simulink model "VFM_linecut_exp"  (R2025a)
settings: Solver=FixedStepAuto  StartTime=0.0  StopTime=t_end+t_sim_start  FixedStep=Ts  RelTol=1e-3
InitFcn:
  | run VFMPara_exp.m
values from neighbouring files (symbols this model uses):
  Cf = 0.0083    [GFMPara.m]    (also in GFMPara_exp.m = 0.0249; VFMPara.m = 0.02; VFMPara_exp.m = 0.03)
  dt_sag = t_c    [GFMPara.m]    (also in GFMPara_exp.m; PLLpara.m; VFMPara.m; VFMPara_exp.m)
  f_switching = 20e3    (= 20000)    [GFMPara_exp.m]    (also in PLLpara.m = 10000; VFMPara_exp.m)
  Lc = 1e-9    (= 1e-09)    [GFMPara.m]    (also in GFMPara_exp.m; PLLpara.m; VFMPara.m; VFMPara_exp.m)
  Lf = 0.0592    [GFMPara.m]    (also in GFMPara_exp.m; PLLpara.m = 0.05; VFMPara.m = 0.05; VFMPara_exp.m = 0.05)
  Lg1 = X1    [PLLpara.m]    (also in VFMPara.m; VFMPara_exp.m)
  Lgg = Xgg    [PLLpara.m]    (also in VFMPara.m; VFMPara_exp.m)
  m_gfm = 1/D    [GFMPara.m]    (also in GFMPara_exp.m)
  Rf = 1e-3    (= 0.001)    [PLLpara.m]
  Rg1 = R1    [PLLpara.m]    (also in VFMPara.m; VFMPara_exp.m = 4*R1/5)
  Rgg = Rgg    [PLLpara.m]    (also in VFMPara.m; VFMPara_exp.m)
  Sbase = 1    [GFMPara.m]    (also in GFMPara_exp.m; PLLpara.m; VFMPara.m; VFMPara_exp.m)
  Scale_ki_v = 20    [GFMPara.m]    (also in GFMPara_exp.m; VFMPara.m; VFMPara_exp.m)
  t0 = t_sim_start +t_start    [PLLpara.m]    (also in VFMPara_exp.m)
  t0_sag = t_sim_start +t_start    [GFMPara.m]    (also in GFMPara_exp.m; PLLpara.m = 20; VFMPara.m; VFMPara_exp.m = 20)
  tc = t_c    [PLLpara.m]    (also in VFMPara_exp.m)
  Tc = 1/f_switching    (= 5e-05)    [GFMPara_exp.m]    (also in PLLpara.m = 0.0001; VFMPara_exp.m)
  Ts = 1/Fs    (= 1e-05)    [GFMPara.m]    (also in GFMPara_exp.m = 1e-06; PLLpara.m = 1e-06; VFMPara.m = 5e-06; VFMPara_exp.m = 1e-06)
  v_sag = Ug_fault    [GFMPara.m]    (also in GFMPara_exp.m; PLLpara.m; VFMPara.m; VFMPara_exp.m)
  Vbase = 1    [GFMPara.m]    (also in GFMPara_exp.m; PLLpara.m; VFMPara.m; VFMPara_exp.m)
  Vdc = 2.5    [PLLpara.m]
  Vdc_ref = 2.5    [GFMPara_exp.m]
  w_droop = D/J    [GFMPara.m]    (also in GFMPara_exp.m; VFMPara.m = 314.159265359; VFMPara_exp.m = 314.159265359)
  w_i_GFM = 2000*2*pi    (= 12566.3706144)    [GFMPara.m]    (also in GFMPara_exp.m = 9424.77796077; VFMPara.m = 9424.77796077; VFMPara_exp.m = 9424.77796077)
  w_v_GFM = 800 *2*pi    (= 5026.54824574)    [GFMPara.m]    (also in GFMPara_exp.m = 3141.59265359; VFMPara.m = 3141.59265359; VFMPara_exp.m = 3141.59265359)
  Wbase = 2*pi*50    (= 314.159265359)    [GFMPara.m]    (also in GFMPara_exp.m; PLLpara.m; VFMPara.m; VFMPara_exp.m)
  Zbase = Vbase/Ibase    (= 1)    [GFMPara.m]    (also in GFMPara_exp.m; PLLpara.m; VFMPara.m; VFMPara_exp.m)
undefined symbols (not defined in the file or in its folder): DiscIntNeverNeededParam, dspblkCoreblockFVToolHelper, gcbh, initial, Kip, Kpp, Pin, Ws, Y_dc
libraries: spsVoltageMeasurementLib x51, spsCurrentMeasurementLib x48, spsThreePhaseSeriesRLCBranchLib x14, spsControlledVoltageSourceLib x9, spsSeriesRLCBranchLib x8, spsIdealSwitchLib x7, simulink x6, spsThreePhaseBreakerLib x4, spsDCVoltageSourceLib x4, spsControlledCurrentSourceLib x3, spsDiodeLib x3, spsHalfBridgeConverterLib x3
(part 2 of 4)

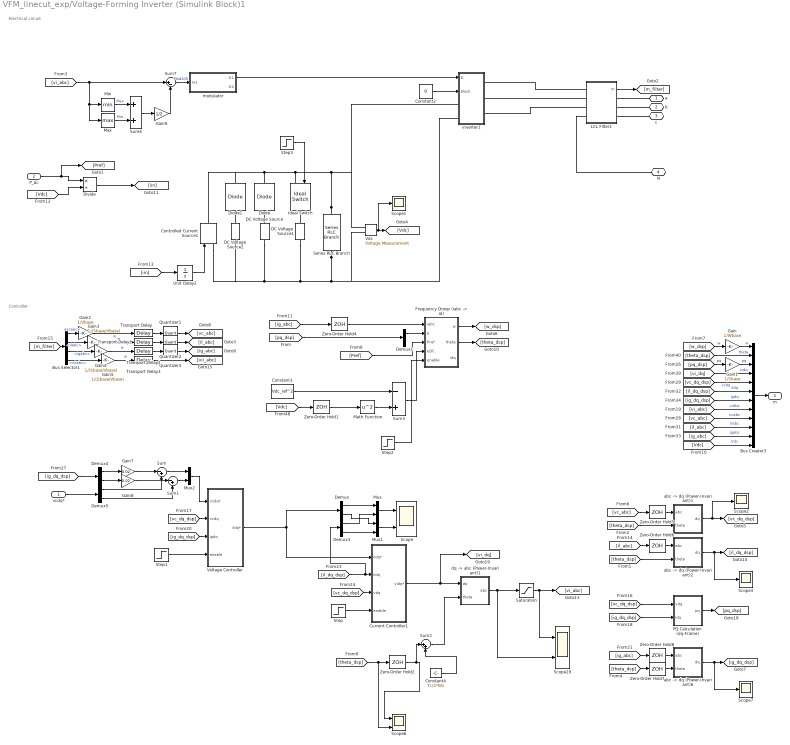
== system VFM_linecut_exp/Voltage-Forming Inverter (Simulink Block)1 ==
  note: Controller
  note: Electrical circuit
  vcdq* : Inport
  P_dc : Inport  Port=2
  Bus Creator3 : BusCreator  Inputs=12
  Bus Selector1 : BusSelector  OutputSignals=vcabc,ilabc,igabc,viiabc
  Constant2 : Constant  Value=0
  Constant3 : Constant  Value=Vdc_ref^2
  Constant4 : Constant  Value=Tc/2*Ws
  Controlled Current Source1 : spsControlledCurrentSourceLib/Controlled Current Source  Initialize=on  Source_Type=AC  Amplitude=0  Phase=0  Frequency=0  Measurements=None
  Current Controller1 : Subsystem  mask{Ts=Tc, Wbase=Wbase, Lf=Lf/Wbase, Kg=0, Kp=w_i*Lf/Wbase*1.5, Ki=w_i*w_i/4*Lf/Wbase, vdmax=Vdc/sqrt(2), vqmax=Vdc/sqrt(2), Kcd=0, Kic=0}
      mask prompts: Ts "Sampling Time (s)"; Wbase "Base Angular Frequency (rad/s)"; Lf "Inductance"; Kg "Estimator Gain"; Kp "Proportional Gain"; Ki "Integral Gain"; vdmax "Voltage D Limit"; vqmax "Voltage Q Limit"; Kcd "Cross Decoupling Gain"; Kic "Capacitor Current Gain"
  DC Voltage Source : spsDCVoltageSourceLib/DC Voltage Source  Amplitude=3.25  Measurements=None
  DC Voltage Source1 : spsDCVoltageSourceLib/DC Voltage Source  Amplitude=2.5  Measurements=None
  DC Voltage Source2 : spsDCVoltageSourceLib/DC Voltage Source  Amplitude=2  Measurements=None
  Demux{,1,3..5} (5 alike) : Demux  Outputs=2
  Diode : spsDiodeLib/Diode  Ron=0.01  Lon=0  Vf=0  IC=0  UseSnubber=0  Rs=1e6  Cs=inf  Measurements=off
  Diode1 : spsDiodeLib/Diode  Ron=0.01  Lon=0  Vf=0  IC=0  UseSnubber=0  Rs=1e6  Cs=inf  Measurements=off
  Divide : Product  Inputs=*/
  "Frequency Droop (iabc -> id)" : Subsystem  AncestorBlock=|  mask{Ts=Tc, Sbase=Sbase, Vbase=Vbase, Wbase=Wbase, m=m, w_tau=w_droop, theta0=0, i0=Pin, w0=1}
      | SimplexPS/Frequency Droop
      | (iabc -> id)
      mask prompts: Ts "Ts (s), samping period"; Sbase "Sbase (VA), base power"; Vbase "Vbase (V), base voltage"; Wbase "Wbase (rad/s), base angular frequency"; m "m (pu), droop gain"; w_tau "w_tau (rad/s), low-pass filter bandwidth"; theta0 "theta0 (rad), initial angle"; i0 "i0 (pu), current setting point"; w0 "w0 (pu), frequency setting point"
  Gain : Gain  Gain=1/Wbase
  Gain1 : Gain  Gain=1/Sbase
  Gain2 : Gain  Gain=1/Vbase
  Gain3 : Gain  Gain=1/(Sbase/Vbase)
  Gain4 : Gain  Gain=1/(Sbase/Vbase)
  Gain5 : Gain  Gain=1/(Sbase/Vbase)
  Gain7 : Gain  Gain=0.02
  Gain8 : Gain  Gain=0.02
  Gain9 : Gain  Gain=1/2
  Ideal Switch : spsIdealSwitchLib/Ideal Switch  Ron=0.001  Lon=0  IC=0  Rs=1e8  Cs=inf  Measurements=off
  LCL Filter1 : Subsystem  mask{Lf=Lf*(Vbase^2/Sbase)/Wbase, Rf=Lf*(Vbase^2/Sbase)*2e-6, Lc=1e-9*(Vbase^2/Sbase)/Wbase, Rc=1e-9*(Vbase^2/Sbase), Cf=Cf*(Sbase/Vbase^2)/Wbase, Rd=1e-3*(Vbase^2/Sbase)}
      mask prompts: Lf "Lf (H)"; Rf "Rf (Ohm)"; Lc "Lc (H)"; Rc "Rc (Ohm)"; Cf "Cf (F)"; Rd "Rd (Ohm)"
  Math Function : Math  Operator=square
  Max : MinMax  Function=max
  Min : MinMax
  Mux : Mux  Inputs=2
  Mux1 : Mux  Inputs=2
  Mux2 : Mux  Inputs=2
  PQ Calculation (dq-Frame) : Subsystem
  Quantizer1 : Quantizer  QuantizationInterval=5/4095
  Quantizer2 : Quantizer  QuantizationInterval=5/4095
  Quantizer3 : Quantizer  QuantizationInterval=5/4095
  Saturation : Saturate  UpperLimit=Vdc_ref/sqrt(3)  LowerLimit=-Vdc_ref/sqrt(3)
  Scope : Scope  NumInputPorts=2
      settings: ActiveDisplayYMinimum=-2.0933971200476993  ActiveDisplayYMaximum=2.0858879407185071  DataLoggingVariableName=ScopeData4
  Scope{1..3,7} (4 alike) : Scope
      Scope1 settings: ActiveDisplayYMinimum=2.0924827237669028  ActiveDisplayYMaximum=4.2567675140943511  DataLoggingVariableName=ScopeData8
      Scope2 settings: ActiveDisplayYMinimum=-2.4523  ActiveDisplayYMaximum=2.43362  DataLoggingVariableName=ScopeData9
      Scope3 settings: ActiveDisplayYMinimum=0.94065  ActiveDisplayYMaximum=1.03256  DataLoggingVariableName=ScopeData11
      Scope7 settings: ActiveDisplayYMinimum=-0.01957  ActiveDisplayYMaximum=0.02954  DataLoggingVariableName=ScopeData10
  Scope29 : Scope  NumInputPorts=2
      settings: ActiveDisplayYMinimum=-28.9342  ActiveDisplayYMaximum=29.0712  DataLoggingVariableName=ScopeData14
  Scope6 : Scope  NumInputPorts=2
      settings: ActiveDisplayYMinimum=2.25613  ActiveDisplayYMaximum=3.2738  DataLoggingVariableName=ScopeData16
  Series RLC Branch : spsSeriesRLCBranchLib/Series RLC Branch  LConnTagsString=__new0  RConnTagsString=__new0  BranchType=RC  Resistance=1e-10*(Vbase^2/Sbase)  Inductance=1e-3  SetiL0=off  InitialCurrent=0  Capacitance=Y_dc*(Sbase/Vbase^2)/Wbase  Setx0=on  InitialVoltage=Vdc_ref  Measurements=None
  Step : Step  Time=0.1  SampleTime=0
  Step1 : Step  Time=0.1  SampleTime=0
  Step2 : Step  Time=0.1  SampleTime=0
  Step3 : Step  Time=0.1  Before=1  After=0  SampleTime=0
  Sum : Sum  Inputs=|-+
  Sum1 : Sum  Inputs=|-+
  Sum2 : Sum  Inputs=|++  InputSameDT=on  SaturateOnIntegerOverflow=on  OutDataTypeStr=Inherit: Same as first input
  Sum3 : Sum  Inputs=-+
  Sum6 : Sum  InputSameDT=on  SaturateOnIntegerOverflow=on  OutDataTypeStr=Inherit: Same as first input
  Sum7 : Sum  Inputs=|+-  InputSameDT=on  SaturateOnIntegerOverflow=on  OutDataTypeStr=Inherit: Same as first input
  Transport Delay{,1..3} (4 alike) : TransportDelay  DelayTime=6e-6
  Unit Delay2 : UnitDelay  SampleTime=-1  HasFrameUpgradeWarning=on
  Vdc : spsVoltageMeasurementLib/Voltage Measurement  PhasorSimulation=off  OutputType=Complex  PSBequivalent=0
  Voltage Controller : Subsystem  mask{Ts=Tc, Wbase=Wbase, Cf=Cf/Wbase, Kg=0, Kp=w_v*Cf/Wbase, Ki=w_v*w_v/4*Cf/Wbase*Scale_ki_v, xdmax=inf, xqmax=inf, Kcd=0}
      mask prompts: Ts "Sampling Time (s)"; Wbase "Base Angular Frequency (rad/s)"; Cf "Capacitance"; Kg "Estimator Gain"; Kp "Proportional Gain"; Ki "Integral Gain"; xdmax "Current D Limit"; xqmax "Current Q Limit"; Kcd "Cross Decoupling Gain"
  Zero-Order Hold{1..2,4..8} (7 alike) : ZeroOrderHold  SampleTime=Tc
  "abc -> dq (Power-Invariant)1" : Subsystem  AncestorBlock=|
      | SimplusGT/abc -> dq
      | (Power-Invariant)
  "abc -> dq (Power-Invariant)2" : Subsystem  AncestorBlock=|
      | SimplusGT/abc -> dq
      | (Power-Invariant)
  "abc -> dq (Power-Invariant)6" : Subsystem  AncestorBlock=|
      | SimplusGT/abc -> dq
      | (Power-Invariant)
  "dq -> abc (Power-Invariant)1" : Subsystem  AncestorBlock=|
      | SimplusGT/dq -> abc
      | (Power-Invariant)
  inverter1 : Subsystem
  modulator : Subsystem
  a : PMIOPort  Side=Right
  b : PMIOPort  Port=2  Side=Right
  c : PMIOPort  Port=3  Side=Right
  N : PMIOPort  Port=4  Side=Right
  m : Outport
  wires:
  [ig_abc] -> Bus Creator3/11  "igabc"
  [il_abc] -> Bus Creator3/10  "ilabc"
  [vc_abc] -> Bus Creator3/9  "vcabc"
  [vi_abc] -> Bus Creator3/8  "viabc"
  [ig_dq_dsp] -> Bus Creator3/7  "igdq"
  [il_dq_dsp] -> Bus Creator3/6  "ildq"
  [vc_dq_dsp] -> Bus Creator3/5  "vcdq"
  [vi_dq] -> Bus Creator3/4  "vidq"
  Gain1/1 -> Bus Creator3/3  "pq"
  [theta_dsp] -> Bus Creator3/2  "theta"
  Gain/1 -> Bus Creator3/1  "w"
  [pq_dsp] -> Gain1/1  "pq"
  [w_dsp] -> Gain/1  "w"
  [ig_abc] -> Zero-Order Hold4/1
  [ig_dq_dsp] -> PQ Calculation (dq-Frame)/2(idq)
  PQ Calculation (dq-Frame)/1(pq) -> [pq_dsp]
  [vc_dq_dsp] -> PQ Calculation (dq-Frame)/1(vdq)
  "Frequency Droop (iabc -> id)"/1(w) -> [w_dsp]
  "Frequency Droop (iabc -> id)"/2(theta) -> [theta_dsp]
  Bus Creator3/1 -> m/1
  Demux1/1 -> "Frequency Droop (iabc -> id)"/2(p)
  [pq_dsp] -> Demux1/1
  Bus Selector1/3 -> Gain4/1  "<igabc>"
  Bus Selector1/2 -> Gain3/1  "<ilabc>"
  Bus Selector1/1 -> Gain2/1  "<vcabc>"
  Gain4/1 -> Transport Delay2/1  "w"
  [m_filter] -> Bus Selector1/1
  Gain2/1 -> Transport Delay/1  "w"
  Gain3/1 -> Transport Delay1/1  "w"
  P_dc/1 -> [Pref], Divide/1
  Vdc/1 -> Scope1/1, [Vdc]
  [iin] -> Unit Delay2/1
  LCL Filter1/1(m) -> [m_filter]
  Divide/1 -> [iin]
  Unit Delay2/1 -> Controlled Current Source1/1
  [Vdc] -> Divide/2
  [Pref] -> "Frequency Droop (iabc -> id)"/3(Pref)
  Math Function/1 -> Sum3/2
  Constant3/1 -> Sum3/1
  [Vdc] -> Zero-Order Hold1/1
  Sum3/1 -> "Frequency Droop (iabc -> id)"/4(eDC)
  [Vdc] -> Bus Creator3/12  "Vdc"
  Step/1 -> Current Controller1/4(enable)
  Current Controller1/1(vidq*) -> "dq -> abc (Power-Invariant)1"/1(dq), [vi_dq]
  [vc_dq_dsp] -> Voltage Controller/2(vcdq)
  [vc_dq_dsp] -> Current Controller1/3(vdq)
  [il_dq_dsp] -> Current Controller1/2(iIdq), Demux3/1
  [ig_dq_dsp] -> Voltage Controller/3(igdq)
  "dq -> abc (Power-Invariant)1"/1(abc) -> Scope29/2, Saturation/1
  Sum2/1 -> "dq -> abc (Power-Invariant)1"/2(theta)
  Bus Selector1/4 -> Gain5/1  "<viiabc>"
  Gain5/1 -> Transport Delay3/1  "w"
  Mux/1 -> Scope/1
  Mux1/1 -> Scope/2
  Demux/1 -> Mux/1
  Demux3/1 -> Mux/2
  Demux/2 -> Mux1/1
  Demux3/2 -> Mux1/2
  Demux4/1 -> Gain7/1
  [ig_dq_dsp] -> Demux4/1
  vcdq*/1 -> Demux5/1
  Demux4/2 -> Gain8/1
  Gain8/1 -> Sum1/1
  Gain7/1 -> Sum/1
  Demux5/1 -> Sum/2
  Sum/1 -> Mux2/1
  Demux5/2 -> Sum1/2
  Sum1/1 -> Mux2/2
  Mux2/1 -> Voltage Controller/1(vcdq*)
  Sum7/1 -> modulator/1(In1)  "ModA/B"
  Sum6/1 -> Gain9/1
  [vi_abc] -> Sum7/1, Max/1, Min/1
  Max/1 -> Sum6/2  "Min"
  Gain9/1 -> Sum7/2
  Min/1 -> Sum6/1  "Max"
  modulator/1(G1) -> inverter1/1(G)
  Constant2/1 -> inverter1/2(block)
  Transport Delay/1 -> Quantizer1/1
  Transport Delay1/1 -> Quantizer2/1
  Transport Delay2/1 -> Quantizer3/1
  Transport Delay3/1 -> [vii_abc]
  Zero-Order Hold4/1 -> "Frequency Droop (iabc -> id)"/1(iabc)
  [il_abc] -> Zero-Order Hold6/1
  [theta_dsp] -> "abc -> dq (Power-Invariant)1"/2(theta)
  "abc -> dq (Power-Invariant)2"/1(dq) -> Scope3/1, [il_dq_dsp]
  Zero-Order Hold5/1 -> "abc -> dq (Power-Invariant)1"/1(abc)
  Zero-Order Hold6/1 -> "abc -> dq (Power-Invariant)2"/1(abc)
  [vc_abc] -> Zero-Order Hold5/1
  "abc -> dq (Power-Invariant)1"/1(dq) -> Scope2/1, [vc_dq_dsp]
  [theta_dsp] -> "abc -> dq (Power-Invariant)2"/2(theta)
  Zero-Order Hold7/1 -> "abc -> dq (Power-Invariant)6"/2(theta)
  [theta_dsp] -> Zero-Order Hold7/1
  "abc -> dq (Power-Invariant)6"/1(dq) -> Scope7/1, [ig_dq_dsp]
  Zero-Order Hold8/1 -> "abc -> dq (Power-Invariant)6"/1(abc)
  [ig_abc] -> Zero-Order Hold8/1
  Zero-Order Hold1/1 -> Math Function/1
  Saturation/1 -> Scope29/1, [vi_abc]
  [theta_dsp] -> Scope6/2, Zero-Order Hold2/1
  Zero-Order Hold2/1 -> Sum2/1, Scope6/1
  Constant4/1 -> Sum2/2
  Step1/1 -> Voltage Controller/4(enable)
  Voltage Controller/1(ildq*) -> Demux/1, Current Controller1/1(iIdq*)
  Step2/1 -> "Frequency Droop (iabc -> id)"/5(enable)
  Step3/1 -> Ideal Switch/1
  Quantizer1/1 -> [vc_abc]
  Quantizer2/1 -> [il_abc]
  Quantizer3/1 -> [ig_abc]
  connections:
  Series RLC Branch/LConn1 -- Ideal Switch/LConn1 -- Diode1/RConn1 -- Controlled Current Source1/RConn1 -- Diode/LConn1 -- Vdc/LConn1 -- inverter1/LConn1
  N/RConn1 -- LCL Filter1/LConn4
  Series RLC Branch/RConn1 -- DC Voltage Source1/LConn1 -- DC Voltage Source2/LConn1 -- Controlled Current Source1/LConn1 -- DC Voltage Source/LConn1 -- inverter1/LConn2 -- Vdc/LConn2
  LCL Filter1/RConn1 -- a/RConn1
  LCL Filter1/RConn2 -- b/RConn1
  LCL Filter1/RConn3 -- c/RConn1
  DC Voltage Source/RConn1 -- Diode/RConn1
  DC Voltage Source2/RConn1 -- Diode1/LConn1
  LCL Filter1/LConn2 -- inverter1/RConn2
  LCL Filter1/LConn1 -- inverter1/RConn1
  LCL Filter1/LConn3 -- inverter1/RConn3
  DC Voltage Source1/RConn1 -- Ideal Switch/RConn1

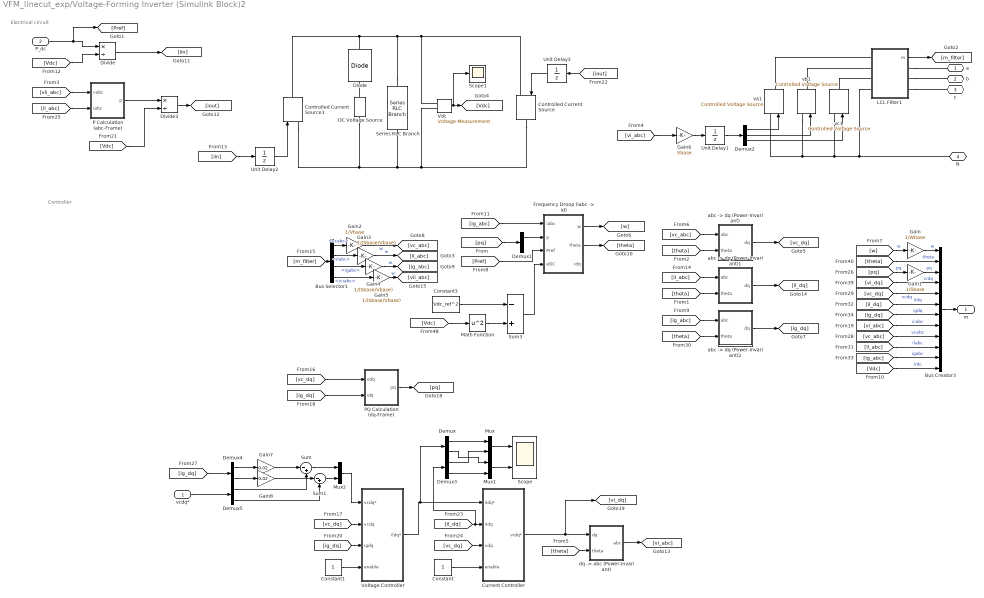
== system VFM_linecut_exp/Voltage-Forming Inverter (Simulink Block)2 ==
  note: Controller
  note: Electrical circuit
  vcdq* : Inport
  P_dc : Inport  Port=2
  Bus Creator3 : BusCreator  Inputs=12
  Bus Selector1 : BusSelector  OutputSignals=vcabc,ilabc,igabc,viiabc
  Constant : Constant
  Constant1 : Constant
  Constant3 : Constant  Value=Vdc_ref^2
  Controlled Current Source : spsControlledCurrentSourceLib/Controlled Current Source  Initialize=on  Source_Type=AC  Amplitude=0  Phase=0  Frequency=0  Measurements=None
  Controlled Current Source1 : spsControlledCurrentSourceLib/Controlled Current Source  Initialize=on  Source_Type=AC  Amplitude=0  Phase=0  Frequency=0  Measurements=None
  Current Controller : Subsystem  mask{Ts=Ts, Wbase=Wbase, Lf=Lf/Wbase, Kg=0, Kp=w_i*Lf/Wbase*2, Ki=w_i*w_i/4*Lf/Wbase, xdmax=inf, xqmax=inf, Kcd=0}
      mask prompts: Ts "Sampling Time (s)"; Wbase "Base Angular Frequency (rad/s)"; Lf "Inductance"; Kg "Estimator Gain"; Kp "Proportional Gain"; Ki "Integral Gain"; xdmax "Voltage D Limit"; xqmax "Voltage Q Limit"; Kcd "Cross Decoupling Gain"
  DC Voltage Source : spsDCVoltageSourceLib/DC Voltage Source  Amplitude=3.25  Measurements=None
  Demux{,1,3..5} (5 alike) : Demux  Outputs=2
  Demux2 : Demux  Outputs=3
  Diode : spsDiodeLib/Diode  Ron=0.01  Lon=0  Vf=0  IC=0  UseSnubber=0  Rs=1e6  Cs=inf  Measurements=off
  Divide : Product  Inputs=*/
  Divide3 : Product  Inputs=*/
  "Frequency Droop (iabc -> id)" : Subsystem  AncestorBlock=|  mask{Ts=Ts, Sbase=Sbase, Vbase=Vbase, Wbase=Wbase, m=m, w_tau=w_droop, theta0=0, i0=Pin, w0=1}
      | SimplexPS/Frequency Droop
      | (iabc -> id)
      mask prompts: Ts "Ts (s), samping period"; Sbase "Sbase (VA), base power"; Vbase "Vbase (V), base voltage"; Wbase "Wbase (rad/s), base angular frequency"; m "m (pu), droop gain"; w_tau "w_tau (rad/s), low-pass filter bandwidth"; theta0 "theta0 (rad), initial angle"; i0 "i0 (pu), current setting point"; w0 "w0 (pu), frequency setting point"
  Gain : Gain  Gain=1/Wbase
  Gain1 : Gain  Gain=1/Sbase
  Gain2 : Gain  Gain=1/Vbase
  Gain3 : Gain  Gain=1/(Sbase/Vbase)
  Gain4 : Gain  Gain=1/(Sbase/Vbase)
  Gain5 : Gain  Gain=1/(Sbase/Vbase)
  Gain6 : Gain  Gain=Vbase
  Gain7 : Gain  Gain=0.02
  Gain8 : Gain  Gain=0.02
  LCL Filter1 : Subsystem  mask{Lf=Lf*(Vbase^2/Sbase)/Wbase, Rf=Lf*(Vbase^2/Sbase)*2e-6, Lc=1e-9*(Vbase^2/Sbase)/Wbase, Rc=1e-9*(Vbase^2/Sbase), Cf=Cf*(Sbase/Vbase^2)/Wbase, Rd=1e-3*(Vbase^2/Sbase)}
      mask prompts: Lf "Lf (H)"; Rf "Rf (Ohm)"; Lc "Lc (H)"; Rc "Rc (Ohm)"; Cf "Cf (F)"; Rd "Rd (Ohm)"
  Math Function : Math  Operator=square
  Mux : Mux  Inputs=2
  Mux1 : Mux  Inputs=2
  Mux2 : Mux  Inputs=2
  P Calculation (abc-Frame) : Subsystem
  PQ Calculation (dq-Frame) : Subsystem
  Scope : Scope  NumInputPorts=2
      settings: ActiveDisplayYMinimum=-0.33464461434412296  ActiveDisplayYMaximum=1.613093583112561  DataLoggingVariableName=ScopeData4
  Scope1 : Scope
      settings: ActiveDisplayYMinimum=2.0924827237669028  ActiveDisplayYMaximum=4.2567675140943511  DataLoggingVariableName=ScopeData8
  Series RLC Branch : spsSeriesRLCBranchLib/Series RLC Branch  LConnTagsString=__new0  RConnTagsString=__new0  BranchType=RC  Resistance=1e-10*(Vbase^2/Sbase)  Inductance=1e-3  SetiL0=off  InitialCurrent=0  Capacitance=Y_dc*(Sbase/Vbase^2)/Wbase  Setx0=on  InitialVoltage=Vdc_ref  Measurements=None
  Sum : Sum  Inputs=|-+
  Sum1 : Sum  Inputs=|-+
  Sum3 : Sum  Inputs=-+
  Unit Delay1 : UnitDelay  SampleTime=Ts  HasFrameUpgradeWarning=on
  Unit Delay2 : UnitDelay  SampleTime=-1  HasFrameUpgradeWarning=on
  Unit Delay3 : UnitDelay  SampleTime=-1  HasFrameUpgradeWarning=on
  Vdc : spsVoltageMeasurementLib/Voltage Measurement  PhasorSimulation=off  OutputType=Complex  PSBequivalent=0
  Voltage Controller : Subsystem  mask{Ts=Ts, Wbase=Wbase, Cf=Cf/Wbase, Kg=0, Kp=w_v*Cf/Wbase, Ki=w_v*w_v/4*Cf/Wbase*Scale_ki_v, xdmax=inf, xqmax=inf, Kcd=0}
      mask prompts: Ts "Sampling Time (s)"; Wbase "Base Angular Frequency (rad/s)"; Cf "Capacitance"; Kg "Estimator Gain"; Kp "Proportional Gain"; Ki "Integral Gain"; xdmax "Current D Limit"; xqmax "Current Q Limit"; Kcd "Cross Decoupling Gain"
  "abc -> dq (Power-Invariant)" : Subsystem
  "abc -> dq (Power-Invariant)1" : Subsystem
  "abc -> dq (Power-Invariant)2" : Subsystem
  "dq -> abc (Power-Invariant)" : Subsystem
  va1 : spsControlledVoltageSourceLib/Controlled Voltage Source  Initialize=on  Source_Type=AC  Amplitude=0  Phase=0  Frequency=0  Measurements=None
  vb1 : spsControlledVoltageSourceLib/Controlled Voltage Source  Initialize=on  Source_Type=AC  Amplitude=0  Phase=0  Frequency=0  Measurements=None
  vc1 : spsControlledVoltageSourceLib/Controlled Voltage Source  Initialize=on  Source_Type=AC  Amplitude=0  Phase=0  Frequency=0  Measurements=None
  a : PMIOPort  Side=Right
  b : PMIOPort  Port=2  Side=Right
  c : PMIOPort  Port=3  Side=Right
  N : PMIOPort  Port=4  Side=Right
  m : Outport
  wires:
  [ig_abc] -> Bus Creator3/11  "igabc"
  [il_abc] -> Bus Creator3/10  "ilabc"
  [vc_abc] -> Bus Creator3/9  "vcabc"
  [vi_abc] -> Bus Creator3/8  "viabc"
  [ig_dq] -> Bus Creator3/7  "igdq"
  [il_dq] -> Bus Creator3/6  "ildq"
  [vc_dq] -> Bus Creator3/5  "vcdq"
  [vi_dq] -> Bus Creator3/4  "vidq"
  Gain1/1 -> Bus Creator3/3  "pq"
  [theta] -> Bus Creator3/2  "theta"
  Gain/1 -> Bus Creator3/1  "w"
  [pq] -> Gain1/1  "pq"
  [w] -> Gain/1  "w"
  "abc -> dq (Power-Invariant)1"/1(dq) -> [il_dq]
  "abc -> dq (Power-Invariant)2"/1(dq) -> [ig_dq]
  "abc -> dq (Power-Invariant)"/1(dq) -> [vc_dq]
  [ig_abc] -> "Frequency Droop (iabc -> id)"/1(iabc)
  [ig_dq] -> PQ Calculation (dq-Frame)/2(idq)
  PQ Calculation (dq-Frame)/1(pq) -> [pq]
  [vc_dq] -> PQ Calculation (dq-Frame)/1(vdq)
  "Frequency Droop (iabc -> id)"/1(w) -> [w]
  "Frequency Droop (iabc -> id)"/2(theta) -> [theta]
  [theta] -> "abc -> dq (Power-Invariant)2"/2(theta)
  [ig_abc] -> "abc -> dq (Power-Invariant)2"/1(abc)
  [il_abc] -> "abc -> dq (Power-Invariant)1"/1(abc)
  [vc_abc] -> "abc -> dq (Power-Invariant)"/1(abc)
  [theta] -> "abc -> dq (Power-Invariant)1"/2(theta)
  [theta] -> "abc -> dq (Power-Invariant)"/2(theta)
  Bus Creator3/1 -> m/1
  Demux1/1 -> "Frequency Droop (iabc -> id)"/2(p)
  [pq] -> Demux1/1
  Bus Selector1/3 -> Gain4/1  "<igabc>"
  Bus Selector1/2 -> Gain3/1  "<ilabc>"
  Bus Selector1/1 -> Gain2/1  "<vcabc>"
  Gain4/1 -> [ig_abc]  "w"
  [m_filter] -> Bus Selector1/1
  Gain2/1 -> [vc_abc]  "w"
  Gain3/1 -> [il_abc]  "w"
  P_dc/1 -> [Pref], Divide/1
  Vdc/1 -> Scope1/1, [Vdc]
  [iout] -> Unit Delay3/1
  Divide3/1 -> [iout]
  [iin] -> Unit Delay2/1
  LCL Filter1/1(m) -> [m_filter]
  Divide/1 -> [iin]
  Demux2/2 -> vb1/1
  Gain6/1 -> Unit Delay1/1
  Unit Delay3/1 -> Controlled Current Source/1
  Demux2/3 -> vc1/1
  Unit Delay1/1 -> Demux2/1
  Unit Delay2/1 -> Controlled Current Source1/1
  Demux2/1 -> va1/1
  [Vdc] -> Divide3/2
  [Vdc] -> Divide/2
  [Pref] -> "Frequency Droop (iabc -> id)"/3(Pref)
  Math Function/1 -> Sum3/2
  Constant3/1 -> Sum3/1
  [Vdc] -> Math Function/1
  Sum3/1 -> "Frequency Droop (iabc -> id)"/4(eDC)
  [Vdc] -> Bus Creator3/12  "Vdc"
  [vi_abc] -> Gain6/1
  Constant/1 -> Current Controller/4(enable)
  Current Controller/1(vidq*) -> [vi_dq], "dq -> abc (Power-Invariant)"/1(dq)
  [vc_dq] -> Voltage Controller/2(vcdq)
  [vc_dq] -> Current Controller/3(vdq)
  [il_dq] -> Demux3/1, Current Controller/2(iIdq)
  [ig_dq] -> Voltage Controller/3(igdq)
  Voltage Controller/1(ildq*) -> Demux/1, Current Controller/1(iIdq*)
  Constant1/1 -> Voltage Controller/4(enable)
  "dq -> abc (Power-Invariant)"/1(abc) -> [vi_abc]
  [theta] -> "dq -> abc (Power-Invariant)"/2(theta)
  Bus Selector1/4 -> Gain5/1  "<viiabc>"
  Gain5/1 -> [vii_abc]  "w"
  P Calculation (abc-Frame)/1(p) -> Divide3/1
  [vii_abc] -> P Calculation (abc-Frame)/1(vabc)
  [il_abc] -> P Calculation (abc-Frame)/2(iabc)
  Mux/1 -> Scope/1
  Mux1/1 -> Scope/2
  Demux/1 -> Mux/1
  Demux3/1 -> Mux/2
  Demux/2 -> Mux1/1
  Demux3/2 -> Mux1/2
  Demux4/1 -> Gain7/1
  [ig_dq] -> Demux4/1
  vcdq*/1 -> Demux5/1
  Demux4/2 -> Gain8/1
  Gain8/1 -> Sum1/1
  Gain7/1 -> Sum/1
  Demux5/1 -> Sum/2
  Sum/1 -> Mux2/1
  Demux5/2 -> Sum1/2
  Sum1/1 -> Mux2/2
  Mux2/1 -> Voltage Controller/1(vcdq*)
  connections:
  Series RLC Branch/LConn1 -- Controlled Current Source1/RConn1 -- Diode/LConn1 -- Vdc/LConn1 -- Controlled Current Source/LConn1
  va1/LConn1 -- LCL Filter1/LConn4 -- N/RConn1 -- vc1/LConn1 -- vb1/LConn1
  Series RLC Branch/RConn1 -- Controlled Current Source1/LConn1 -- DC Voltage Source/LConn1 -- Controlled Current Source/RConn1 -- Vdc/LConn2
  LCL Filter1/LConn2 -- vb1/RConn1
  LCL Filter1/RConn1 -- a/RConn1
  LCL Filter1/LConn3 -- vc1/RConn1
  LCL Filter1/LConn1 -- va1/RConn1
  LCL Filter1/RConn2 -- b/RConn1
  LCL Filter1/RConn3 -- c/RConn1
  DC Voltage Source/RConn1 -- Diode/RConn1

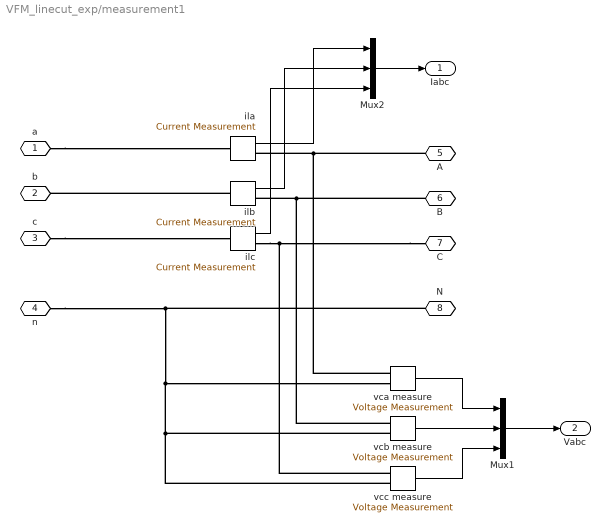
== system VFM_linecut_exp/measurement1 ==
  Mux1 : Mux  Inputs=3
  Mux2 : Mux  Inputs=3
  ila : spsCurrentMeasurementLib/Current Measurement  PhasorSimulation=off  OutputType=Complex  PSBequivalent=0
  ilb : spsCurrentMeasurementLib/Current Measurement  PhasorSimulation=off  OutputType=Complex  PSBequivalent=0
  ilc : spsCurrentMeasurementLib/Current Measurement  PhasorSimulation=off  OutputType=Complex  PSBequivalent=0
  vca measure : spsVoltageMeasurementLib/Voltage Measurement  PhasorSimulation=off  OutputType=Complex  PSBequivalent=0
  vcb measure : spsVoltageMeasurementLib/Voltage Measurement  PhasorSimulation=off  OutputType=Complex  PSBequivalent=0
  vcc measure : spsVoltageMeasurementLib/Voltage Measurement  PhasorSimulation=off  OutputType=Complex  PSBequivalent=0
  a : PMIOPort  Side=Left
  b : PMIOPort  Port=2  Side=Left
  c : PMIOPort  Port=3  Side=Left
  n : PMIOPort  Port=4  Side=Left
  A : PMIOPort  Port=5  Side=Right
  B : PMIOPort  Port=6  Side=Right
  C : PMIOPort  Port=7  Side=Right
  N : PMIOPort  Port=8  Side=Right
  Iabc : Outport
  Vabc : Outport  Port=2
  wires:
  ila/1 -> Mux2/1
  ilb/1 -> Mux2/2
  ilc/1 -> Mux2/3
  Mux2/1 -> Iabc/1
  vcb measure/1 -> Mux1/2
  vca measure/1 -> Mux1/1
  vcc measure/1 -> Mux1/3
  Mux1/1 -> Vabc/1
  connections:
  a/RConn1 -- ila/LConn1
  ila/RConn1 -- A/RConn1 -- vca measure/LConn1
  ilb/LConn1 -- b/RConn1
  ilb/RConn1 -- B/RConn1 -- vcb measure/LConn1
  c/RConn1 -- ilc/LConn1
  C/RConn1 -- ilc/RConn1 -- vcc measure/LConn1
  n/RConn1 -- vcc measure/LConn2 -- vcb measure/LConn2 -- vca measure/LConn2 -- N/RConn1

== system VFM_linecut_exp/measurement11 ==
  Mux1 : Mux  Inputs=3
  Mux2 : Mux  Inputs=3
  ila : spsCurrentMeasurementLib/Current Measurement  PhasorSimulation=off  OutputType=Complex  PSBequivalent=0
  ilb : spsCurrentMeasurementLib/Current Measurement  PhasorSimulation=off  OutputType=Complex  PSBequivalent=0
  ilc : spsCurrentMeasurementLib/Current Measurement  PhasorSimulation=off  OutputType=Complex  PSBequivalent=0
  vca measure : spsVoltageMeasurementLib/Voltage Measurement  PhasorSimulation=off  OutputType=Complex  PSBequivalent=0
  vcb measure : spsVoltageMeasurementLib/Voltage Measurement  PhasorSimulation=off  OutputType=Complex  PSBequivalent=0
  vcc measure : spsVoltageMeasurementLib/Voltage Measurement  PhasorSimulation=off  OutputType=Complex  PSBequivalent=0
  a : PMIOPort  Side=Left
  b : PMIOPort  Port=2  Side=Left
  c : PMIOPort  Port=3  Side=Left
  n : PMIOPort  Port=4  Side=Left
  A : PMIOPort  Port=5  Side=Right
  B : PMIOPort  Port=6  Side=Right
  C : PMIOPort  Port=7  Side=Right
  N : PMIOPort  Port=8  Side=Right
  Iabc : Outport
  Vabc : Outport  Port=2
  wires:
  ila/1 -> Mux2/1
  ilb/1 -> Mux2/2
  ilc/1 -> Mux2/3
  Mux2/1 -> Iabc/1
  vcb measure/1 -> Mux1/2
  vca measure/1 -> Mux1/1
  vcc measure/1 -> Mux1/3
  Mux1/1 -> Vabc/1
  connections:
  a/RConn1 -- ila/LConn1
  ila/RConn1 -- A/RConn1 -- vca measure/LConn1
  ilb/LConn1 -- b/RConn1
  ilb/RConn1 -- B/RConn1 -- vcb measure/LConn1
  c/RConn1 -- ilc/LConn1
  C/RConn1 -- ilc/RConn1 -- vcc measure/LConn1
  n/RConn1 -- vcc measure/LConn2 -- vcb measure/LConn2 -- vca measure/LConn2 -- N/RConn1

== system VFM_linecut_exp/measurement12 ==
  Mux1 : Mux  Inputs=3
  Mux2 : Mux  Inputs=3
  ila : spsCurrentMeasurementLib/Current Measurement  PhasorSimulation=off  OutputType=Complex  PSBequivalent=0
  ilb : spsCurrentMeasurementLib/Current Measurement  PhasorSimulation=off  OutputType=Complex  PSBequivalent=0
  ilc : spsCurrentMeasurementLib/Current Measurement  PhasorSimulation=off  OutputType=Complex  PSBequivalent=0
  vca measure : spsVoltageMeasurementLib/Voltage Measurement  PhasorSimulation=off  OutputType=Complex  PSBequivalent=0
  vcb measure : spsVoltageMeasurementLib/Voltage Measurement  PhasorSimulation=off  OutputType=Complex  PSBequivalent=0
  vcc measure : spsVoltageMeasurementLib/Voltage Measurement  PhasorSimulation=off  OutputType=Complex  PSBequivalent=0
  a : PMIOPort  Side=Left
  b : PMIOPort  Port=2  Side=Left
  c : PMIOPort  Port=3  Side=Left
  n : PMIOPort  Port=4  Side=Left
  A : PMIOPort  Port=5  Side=Right
  B : PMIOPort  Port=6  Side=Right
  C : PMIOPort  Port=7  Side=Right
  N : PMIOPort  Port=8  Side=Right
  Iabc : Outport
  Vabc : Outport  Port=2
  wires:
  ila/1 -> Mux2/1
  ilb/1 -> Mux2/2
  ilc/1 -> Mux2/3
  Mux2/1 -> Iabc/1
  vcb measure/1 -> Mux1/2
  vca measure/1 -> Mux1/1
  vcc measure/1 -> Mux1/3
  Mux1/1 -> Vabc/1
  connections:
  a/RConn1 -- ila/LConn1
  ila/RConn1 -- A/RConn1 -- vca measure/LConn1
  ilb/LConn1 -- b/RConn1
  ilb/RConn1 -- B/RConn1 -- vcb measure/LConn1
  c/RConn1 -- ilc/LConn1
  C/RConn1 -- ilc/RConn1 -- vcc measure/LConn1
  n/RConn1 -- vcc measure/LConn2 -- vcb measure/LConn2 -- vca measure/LConn2 -- N/RConn1

== system VFM_linecut_exp/measurement13 ==
  Mux1 : Mux  Inputs=3
  Mux2 : Mux  Inputs=3
  ila : spsCurrentMeasurementLib/Current Measurement  PhasorSimulation=off  OutputType=Complex  PSBequivalent=0
  ilb : spsCurrentMeasurementLib/Current Measurement  PhasorSimulation=off  OutputType=Complex  PSBequivalent=0
  ilc : spsCurrentMeasurementLib/Current Measurement  PhasorSimulation=off  OutputType=Complex  PSBequivalent=0
  vca measure : spsVoltageMeasurementLib/Voltage Measurement  PhasorSimulation=off  OutputType=Complex  PSBequivalent=0
  vcb measure : spsVoltageMeasurementLib/Voltage Measurement  PhasorSimulation=off  OutputType=Complex  PSBequivalent=0
  vcc measure : spsVoltageMeasurementLib/Voltage Measurement  PhasorSimulation=off  OutputType=Complex  PSBequivalent=0
  a : PMIOPort  Side=Left
  b : PMIOPort  Port=2  Side=Left
  c : PMIOPort  Port=3  Side=Left
  n : PMIOPort  Port=4  Side=Left
  A : PMIOPort  Port=5  Side=Right
  B : PMIOPort  Port=6  Side=Right
  C : PMIOPort  Port=7  Side=Right
  N : PMIOPort  Port=8  Side=Right
  Iabc : Outport
  Vabc : Outport  Port=2
  wires:
  ila/1 -> Mux2/1
  ilb/1 -> Mux2/2
  ilc/1 -> Mux2/3
  Mux2/1 -> Iabc/1
  vcb measure/1 -> Mux1/2
  vca measure/1 -> Mux1/1
  vcc measure/1 -> Mux1/3
  Mux1/1 -> Vabc/1
  connections:
  a/RConn1 -- ila/LConn1
  ila/RConn1 -- A/RConn1 -- vca measure/LConn1
  ilb/LConn1 -- b/RConn1
  ilb/RConn1 -- B/RConn1 -- vcb measure/LConn1
  c/RConn1 -- ilc/LConn1
  C/RConn1 -- ilc/RConn1 -- vcc measure/LConn1
  n/RConn1 -- vcc measure/LConn2 -- vcb measure/LConn2 -- vca measure/LConn2 -- N/RConn1

== system VFM_linecut_exp/measurement14 ==
  Mux1 : Mux  Inputs=3
  Mux2 : Mux  Inputs=3
  ila : spsCurrentMeasurementLib/Current Measurement  PhasorSimulation=off  OutputType=Complex  PSBequivalent=0
  ilb : spsCurrentMeasurementLib/Current Measurement  PhasorSimulation=off  OutputType=Complex  PSBequivalent=0
  ilc : spsCurrentMeasurementLib/Current Measurement  PhasorSimulation=off  OutputType=Complex  PSBequivalent=0
  vca measure : spsVoltageMeasurementLib/Voltage Measurement  PhasorSimulation=off  OutputType=Complex  PSBequivalent=0
  vcb measure : spsVoltageMeasurementLib/Voltage Measurement  PhasorSimulation=off  OutputType=Complex  PSBequivalent=0
  vcc measure : spsVoltageMeasurementLib/Voltage Measurement  PhasorSimulation=off  OutputType=Complex  PSBequivalent=0
  a : PMIOPort  Side=Left
  b : PMIOPort  Port=2  Side=Left
  c : PMIOPort  Port=3  Side=Left
  n : PMIOPort  Port=4  Side=Left
  A : PMIOPort  Port=5  Side=Right
  B : PMIOPort  Port=6  Side=Right
  C : PMIOPort  Port=7  Side=Right
  N : PMIOPort  Port=8  Side=Right
  Iabc : Outport
  Vabc : Outport  Port=2
  wires:
  ila/1 -> Mux2/1
  ilb/1 -> Mux2/2
  ilc/1 -> Mux2/3
  Mux2/1 -> Iabc/1
  vcb measure/1 -> Mux1/2
  vca measure/1 -> Mux1/1
  vcc measure/1 -> Mux1/3
  Mux1/1 -> Vabc/1
  connections:
  a/RConn1 -- ila/LConn1
  ila/RConn1 -- A/RConn1 -- vca measure/LConn1
  ilb/LConn1 -- b/RConn1
  ilb/RConn1 -- B/RConn1 -- vcb measure/LConn1
  c/RConn1 -- ilc/LConn1
  C/RConn1 -- ilc/RConn1 -- vcc measure/LConn1
  n/RConn1 -- vcc measure/LConn2 -- vcb measure/LConn2 -- vca measure/LConn2 -- N/RConn1

== system VFM_linecut_exp/measurement15 ==
  Mux1 : Mux  Inputs=3
  Mux2 : Mux  Inputs=3
  ila : spsCurrentMeasurementLib/Current Measurement  PhasorSimulation=off  OutputType=Complex  PSBequivalent=0
  ilb : spsCurrentMeasurementLib/Current Measurement  PhasorSimulation=off  OutputType=Complex  PSBequivalent=0
  ilc : spsCurrentMeasurementLib/Current Measurement  PhasorSimulation=off  OutputType=Complex  PSBequivalent=0
  vca measure : spsVoltageMeasurementLib/Voltage Measurement  PhasorSimulation=off  OutputType=Complex  PSBequivalent=0
  vcb measure : spsVoltageMeasurementLib/Voltage Measurement  PhasorSimulation=off  OutputType=Complex  PSBequivalent=0
  vcc measure : spsVoltageMeasurementLib/Voltage Measurement  PhasorSimulation=off  OutputType=Complex  PSBequivalent=0
  a : PMIOPort  Side=Left
  b : PMIOPort  Port=2  Side=Left
  c : PMIOPort  Port=3  Side=Left
  n : PMIOPort  Port=4  Side=Left
  A : PMIOPort  Port=5  Side=Right
  B : PMIOPort  Port=6  Side=Right
  C : PMIOPort  Port=7  Side=Right
  N : PMIOPort  Port=8  Side=Right
  Iabc : Outport
  Vabc : Outport  Port=2
  wires:
  ila/1 -> Mux2/1
  ilb/1 -> Mux2/2
  ilc/1 -> Mux2/3
  Mux2/1 -> Iabc/1
  vcb measure/1 -> Mux1/2
  vca measure/1 -> Mux1/1
  vcc measure/1 -> Mux1/3
  Mux1/1 -> Vabc/1
  connections:
  a/RConn1 -- ila/LConn1
  ila/RConn1 -- A/RConn1 -- vca measure/LConn1
  ilb/LConn1 -- b/RConn1
  ilb/RConn1 -- B/RConn1 -- vcb measure/LConn1
  c/RConn1 -- ilc/LConn1
  C/RConn1 -- ilc/RConn1 -- vcc measure/LConn1
  n/RConn1 -- vcc measure/LConn2 -- vcb measure/LConn2 -- vca measure/LConn2 -- N/RConn1

== system VFM_linecut_exp/measurement3 ==
  Mux1 : Mux  Inputs=3
  Mux2 : Mux  Inputs=3
  ila : spsCurrentMeasurementLib/Current Measurement  PhasorSimulation=off  OutputType=Complex  PSBequivalent=0
  ilb : spsCurrentMeasurementLib/Current Measurement  PhasorSimulation=off  OutputType=Complex  PSBequivalent=0
  ilc : spsCurrentMeasurementLib/Current Measurement  PhasorSimulation=off  OutputType=Complex  PSBequivalent=0
  vca measure : spsVoltageMeasurementLib/Voltage Measurement  PhasorSimulation=off  OutputType=Complex  PSBequivalent=0
  vcb measure : spsVoltageMeasurementLib/Voltage Measurement  PhasorSimulation=off  OutputType=Complex  PSBequivalent=0
  vcc measure : spsVoltageMeasurementLib/Voltage Measurement  PhasorSimulation=off  OutputType=Complex  PSBequivalent=0
  a : PMIOPort  Side=Left
  b : PMIOPort  Port=2  Side=Left
  c : PMIOPort  Port=3  Side=Left
  n : PMIOPort  Port=4  Side=Left
  A : PMIOPort  Port=5  Side=Right
  B : PMIOPort  Port=6  Side=Right
  C : PMIOPort  Port=7  Side=Right
  N : PMIOPort  Port=8  Side=Right
  Iabc : Outport
  Vabc : Outport  Port=2
  wires:
  ila/1 -> Mux2/1
  ilb/1 -> Mux2/2
  ilc/1 -> Mux2/3
  Mux2/1 -> Iabc/1
  vcb measure/1 -> Mux1/2
  vca measure/1 -> Mux1/1
  vcc measure/1 -> Mux1/3
  Mux1/1 -> Vabc/1
  connections:
  a/RConn1 -- ila/LConn1
  ila/RConn1 -- A/RConn1 -- vca measure/LConn1
  ilb/LConn1 -- b/RConn1
  ilb/RConn1 -- B/RConn1 -- vcb measure/LConn1
  c/RConn1 -- ilc/LConn1
  C/RConn1 -- ilc/RConn1 -- vcc measure/LConn1
  n/RConn1 -- vcc measure/LConn2 -- vcb measure/LConn2 -- vca measure/LConn2 -- N/RConn1

== system VFM_linecut_exp/measurement4 ==
  Mux1 : Mux  Inputs=3
  Mux2 : Mux  Inputs=3
  ila : spsCurrentMeasurementLib/Current Measurement  PhasorSimulation=off  OutputType=Complex  PSBequivalent=0
  ilb : spsCurrentMeasurementLib/Current Measurement  PhasorSimulation=off  OutputType=Complex  PSBequivalent=0
  ilc : spsCurrentMeasurementLib/Current Measurement  PhasorSimulation=off  OutputType=Complex  PSBequivalent=0
  vca measure : spsVoltageMeasurementLib/Voltage Measurement  PhasorSimulation=off  OutputType=Complex  PSBequivalent=0
  vcb measure : spsVoltageMeasurementLib/Voltage Measurement  PhasorSimulation=off  OutputType=Complex  PSBequivalent=0
  vcc measure : spsVoltageMeasurementLib/Voltage Measurement  PhasorSimulation=off  OutputType=Complex  PSBequivalent=0
  a : PMIOPort  Side=Left
  b : PMIOPort  Port=2  Side=Left
  c : PMIOPort  Port=3  Side=Left
  n : PMIOPort  Port=4  Side=Left
  A : PMIOPort  Port=5  Side=Right
  B : PMIOPort  Port=6  Side=Right
  C : PMIOPort  Port=7  Side=Right
  N : PMIOPort  Port=8  Side=Right
  Iabc : Outport
  Vabc : Outport  Port=2
  wires:
  ila/1 -> Mux2/1
  ilb/1 -> Mux2/2
  ilc/1 -> Mux2/3
  Mux2/1 -> Iabc/1
  vcb measure/1 -> Mux1/2
  vca measure/1 -> Mux1/1
  vcc measure/1 -> Mux1/3
  Mux1/1 -> Vabc/1
  connections:
  a/RConn1 -- ila/LConn1
  ila/RConn1 -- A/RConn1 -- vca measure/LConn1
  ilb/LConn1 -- b/RConn1
  ilb/RConn1 -- B/RConn1 -- vcb measure/LConn1
  c/RConn1 -- ilc/LConn1
  C/RConn1 -- ilc/RConn1 -- vcc measure/LConn1
  n/RConn1 -- vcc measure/LConn2 -- vcb measure/LConn2 -- vca measure/LConn2 -- N/RConn1

== system VFM_linecut_exp/measurement5 ==
  Mux1 : Mux  Inputs=3
  Mux2 : Mux  Inputs=3
  ila : spsCurrentMeasurementLib/Current Measurement  PhasorSimulation=off  OutputType=Complex  PSBequivalent=0
  ilb : spsCurrentMeasurementLib/Current Measurement  PhasorSimulation=off  OutputType=Complex  PSBequivalent=0
  ilc : spsCurrentMeasurementLib/Current Measurement  PhasorSimulation=off  OutputType=Complex  PSBequivalent=0
  vca measure : spsVoltageMeasurementLib/Voltage Measurement  PhasorSimulation=off  OutputType=Complex  PSBequivalent=0
  vcb measure : spsVoltageMeasurementLib/Voltage Measurement  PhasorSimulation=off  OutputType=Complex  PSBequivalent=0
  vcc measure : spsVoltageMeasurementLib/Voltage Measurement  PhasorSimulation=off  OutputType=Complex  PSBequivalent=0
  a : PMIOPort  Side=Left
  b : PMIOPort  Port=2  Side=Left
  c : PMIOPort  Port=3  Side=Left
  n : PMIOPort  Port=4  Side=Left
  A : PMIOPort  Port=5  Side=Right
  B : PMIOPort  Port=6  Side=Right
  C : PMIOPort  Port=7  Side=Right
  N : PMIOPort  Port=8  Side=Right
  Iabc : Outport
  Vabc : Outport  Port=2
  wires:
  ila/1 -> Mux2/1
  ilb/1 -> Mux2/2
  ilc/1 -> Mux2/3
  Mux2/1 -> Iabc/1
  vcb measure/1 -> Mux1/2
  vca measure/1 -> Mux1/1
  vcc measure/1 -> Mux1/3
  Mux1/1 -> Vabc/1
  connections:
  a/RConn1 -- ila/LConn1
  ila/RConn1 -- A/RConn1 -- vca measure/LConn1
  ilb/LConn1 -- b/RConn1
  ilb/RConn1 -- B/RConn1 -- vcb measure/LConn1
  c/RConn1 -- ilc/LConn1
  C/RConn1 -- ilc/RConn1 -- vcc measure/LConn1
  n/RConn1 -- vcc measure/LConn2 -- vcb measure/LConn2 -- vca measure/LConn2 -- N/RConn1

== system VFM_linecut_exp/measurement6 ==
  Mux1 : Mux  Inputs=3
  Mux2 : Mux  Inputs=3
  ila : spsCurrentMeasurementLib/Current Measurement  PhasorSimulation=off  OutputType=Complex  PSBequivalent=0
  ilb : spsCurrentMeasurementLib/Current Measurement  PhasorSimulation=off  OutputType=Complex  PSBequivalent=0
  ilc : spsCurrentMeasurementLib/Current Measurement  PhasorSimulation=off  OutputType=Complex  PSBequivalent=0
  vca measure : spsVoltageMeasurementLib/Voltage Measurement  PhasorSimulation=off  OutputType=Complex  PSBequivalent=0
  vcb measure : spsVoltageMeasurementLib/Voltage Measurement  PhasorSimulation=off  OutputType=Complex  PSBequivalent=0
  vcc measure : spsVoltageMeasurementLib/Voltage Measurement  PhasorSimulation=off  OutputType=Complex  PSBequivalent=0
  a : PMIOPort  Side=Left
  b : PMIOPort  Port=2  Side=Left
  c : PMIOPort  Port=3  Side=Left
  n : PMIOPort  Port=4  Side=Left
  A : PMIOPort  Port=5  Side=Right
  B : PMIOPort  Port=6  Side=Right
  C : PMIOPort  Port=7  Side=Right
  N : PMIOPort  Port=8  Side=Right
  Iabc : Outport
  Vabc : Outport  Port=2
  wires:
  ila/1 -> Mux2/1
  ilb/1 -> Mux2/2
  ilc/1 -> Mux2/3
  Mux2/1 -> Iabc/1
  vcb measure/1 -> Mux1/2
  vca measure/1 -> Mux1/1
  vcc measure/1 -> Mux1/3
  Mux1/1 -> Vabc/1
  connections:
  a/RConn1 -- ila/LConn1
  ila/RConn1 -- A/RConn1 -- vca measure/LConn1
  ilb/LConn1 -- b/RConn1
  ilb/RConn1 -- B/RConn1 -- vcb measure/LConn1
  c/RConn1 -- ilc/LConn1
  C/RConn1 -- ilc/RConn1 -- vcc measure/LConn1
  n/RConn1 -- vcc measure/LConn2 -- vcb measure/LConn2 -- vca measure/LConn2 -- N/RConn1

== system VFM_linecut_exp/AC Infinite Bus (Voltage Type)1/PQ Calculation (dq-Frame)1 ==
  note: Power calculation.
      |
      | Author(s): Yitong Li
      |
      | Notes:
      |
      | The calculation is done in dq frame.
  vdq : Inport
  idq : Inport  Port=2
  Mux : Mux  Inputs=2
  Mux1 : Mux  Inputs=2
  P = vd*id+vq*iq : Fcn  Expr=u[1]*u[3]+u[2]*u[4]
  Q = -vd*iq+vq*id : Fcn  Expr=-u[1]*u[4]+u[2]*u[3]
  pq : Outport
  wires:
  Mux/1 -> pq/1
  P = vd*id+vq*iq/1 -> Mux/1
  vdq/1 -> Mux1/1
  idq/1 -> Mux1/2
  Mux1/1 -> P = vd*id+vq*iq/1, Q = -vd*iq+vq*id/1
  Q = -vd*iq+vq*id/1 -> Mux/2

== system VFM_linecut_exp/AC Infinite Bus (Voltage Type)1/abc -> dq (Power-Invariant)1 ==
  note: Frame transformation from abc to dq.
      |
      | Author(s): Yitong Li
      |
      | Notes:
      |
      | The transformation is power-invariant.
      |
      | theta is the angle that d axis leads a axis.
      |
      | q axis leads d axis by 90 degrees.
  abc : Inport
  theta : Inport  Port=2
  ->d : Fcn  Expr=cos(u(4))*u(1) + cos(u(4)-2/3*pi)*u(2) + cos(u(4)-4/3*pi)*u(3)
  ->q : Fcn  Expr=-sin(u(4))*u(1) - sin(u(4)-2/3*pi)*u(2) - sin(u(4)-4/3*pi)*u(3)
  Gain : Gain  Gain=sqrt(2/3)
  Mux5 : Mux  Inputs=2
  Mux6 : Mux  Inputs=2
  dq : Outport
  wires:
  abc/1 -> Gain/1
  ->d/1 -> Mux6/1
  Gain/1 -> Mux5/1
  theta/1 -> Mux5/2
  ->q/1 -> Mux6/2
  Mux6/1 -> dq/1
  Mux5/1 -> ->d/1, ->q/1

== system VFM_linecut_exp/AC Infinite Bus (Voltage Type)1/dq -> abc (Power-Invariant)1 ==
  note: Frame transformation from dq to abc.
      |
      | Author(s): Yitong Li
      |
      | Notes:
      |
      | The transformation is power-invariant.
      |
      | theta is the angle that dq axis leads alpha/beta axis, specifically, d axis leads alpha axis.
  dq : Inport
  theta : Inport  Port=2
  ->a : Fcn  Expr=cos(u(3))*u(1) - sin(u(3))*u(2)
  ->b : Fcn  Expr=cos(u(3)-2/3*pi)*u(1) - sin(u(3)-2/3*pi)*u(2)
  ->c : Fcn  Expr=cos(u(3)-4/3*pi)*u(1) - sin(u(3)-4/3*pi)*u(2)
  Gain : Gain  Gain=sqrt(2/3)
  Mux5 : Mux  Inputs=2
  Mux6 : Mux  Inputs=3
  abc : Outport
  wires:
  ->b/1 -> Mux6/2
  ->a/1 -> Mux6/1
  Gain/1 -> Mux5/1
  dq/1 -> Gain/1
  ->c/1 -> Mux6/3
  Mux6/1 -> abc/1
  Mux5/1 -> ->b/1, ->a/1, ->c/1
  theta/1 -> Mux5/2

== system VFM_linecut_exp/AC Infinite Bus (Voltage Type)3/PQ Calculation (dq-Frame)1 ==
  note: Power calculation.
      |
      | Author(s): Yitong Li
      |
      | Notes:
      |
      | The calculation is done in dq frame.
  vdq : Inport
  idq : Inport  Port=2
  Mux : Mux  Inputs=2
  Mux1 : Mux  Inputs=2
  P = vd*id+vq*iq : Fcn  Expr=u[1]*u[3]+u[2]*u[4]
  Q = -vd*iq+vq*id : Fcn  Expr=-u[1]*u[4]+u[2]*u[3]
  pq : Outport
  wires:
  Mux/1 -> pq/1
  P = vd*id+vq*iq/1 -> Mux/1
  vdq/1 -> Mux1/1
  idq/1 -> Mux1/2
  Mux1/1 -> P = vd*id+vq*iq/1, Q = -vd*iq+vq*id/1
  Q = -vd*iq+vq*id/1 -> Mux/2

== system VFM_linecut_exp/AC Infinite Bus (Voltage Type)3/abc -> dq (Power-Invariant)1 ==
  note: Frame transformation from abc to dq.
      |
      | Author(s): Yitong Li
      |
      | Notes:
      |
      | The transformation is power-invariant.
      |
      | theta is the angle that d axis leads a axis.
      |
      | q axis leads d axis by 90 degrees.
  abc : Inport
  theta : Inport  Port=2
  ->d : Fcn  Expr=cos(u(4))*u(1) + cos(u(4)-2/3*pi)*u(2) + cos(u(4)-4/3*pi)*u(3)
  ->q : Fcn  Expr=-sin(u(4))*u(1) - sin(u(4)-2/3*pi)*u(2) - sin(u(4)-4/3*pi)*u(3)
  Gain : Gain  Gain=sqrt(2/3)
  Mux5 : Mux  Inputs=2
  Mux6 : Mux  Inputs=2
  dq : Outport
  wires:
  abc/1 -> Gain/1
  ->d/1 -> Mux6/1
  Gain/1 -> Mux5/1
  theta/1 -> Mux5/2
  ->q/1 -> Mux6/2
  Mux6/1 -> dq/1
  Mux5/1 -> ->d/1, ->q/1

== system VFM_linecut_exp/AC Infinite Bus (Voltage Type)3/dq -> abc (Power-Invariant)1 ==
  note: Frame transformation from dq to abc.
      |
      | Author(s): Yitong Li
      |
      | Notes:
      |
      | The transformation is power-invariant.
      |
      | theta is the angle that dq axis leads alpha/beta axis, specifically, d axis leads alpha axis.
  dq : Inport
  theta : Inport  Port=2
  ->a : Fcn  Expr=cos(u(3))*u(1) - sin(u(3))*u(2)
  ->b : Fcn  Expr=cos(u(3)-2/3*pi)*u(1) - sin(u(3)-2/3*pi)*u(2)
  ->c : Fcn  Expr=cos(u(3)-4/3*pi)*u(1) - sin(u(3)-4/3*pi)*u(2)
  Gain : Gain  Gain=sqrt(2/3)
  Mux5 : Mux  Inputs=2
  Mux6 : Mux  Inputs=3
  abc : Outport
  wires:
  ->b/1 -> Mux6/2
  ->a/1 -> Mux6/1
  Gain/1 -> Mux5/1
  dq/1 -> Gain/1
  ->c/1 -> Mux6/3
  Mux6/1 -> abc/1
  Mux5/1 -> ->b/1, ->a/1, ->c/1
  theta/1 -> Mux5/2

== system VFM_linecut_exp/Voltage-Forming Inverter (Simulink Block)1/Current Controller1 ==
  iIdq* : Inport  PortDimensions=2  SampleTime=Tc
  iIdq : Inport  Port=2  SampleTime=Tc
  vdq : Inport  Port=3  SampleTime=Tc
  enable : Inport  Port=4  SampleTime=Tc
  Constant : Constant  Value=Kcd
  Demux1 : Demux  Outputs=2
  Demux2 : Demux  Outputs=2
  Demux3 : Demux  Outputs=2
  Mux : Mux  Inputs=2
  PI-DT-Estimated d : Subsystem  mask{Lf=Lf, Kg=Kg, Kp=Kp, Ki=Ki, xmax=vdmax, xmin=-vdmax, Ts=Ts}
      mask prompts: Lf "Inductance"; Kg "Estimator Gain"; Kp "Proportional Gain"; Ki "Integral Gain"; xmax "Upper Limit"; xmin "Lower Limit"; Ts "Sampling Time"
  PI-DT-Estimated q : Subsystem  mask{Lf=Lf, Kg=Kg, Kp=Kp, Ki=Ki, xmax=vqmax, xmin=-vqmax, Ts=Ts}
      mask prompts: Lf "Inductance"; Kg "Estimator Gain"; Kp "Proportional Gain"; Ki "Integral Gain"; xmax "Upper Limit"; xmin "Lower Limit"; Ts "Sampling Time"
  Product : Product  Inputs=3
  Product1 : Product  Inputs=3
  sum_d : Sum  Inputs=+-
  sum_q : Sum
  wLd : Gain  Gain=Wbase*Lf
  wLq : Gain  Gain=Wbase*Lf
  vidq* : Outport  PortDimensions=2  SampleTime=Tc
  wires:
  Constant/1 -> Product1/1, Product/2
  Product1/1 -> sum_d/2
  wLq/1 -> Product1/2
  Product/1 -> sum_q/1
  wLd/1 -> Product/1
  Demux2/2 -> PI-DT-Estimated q/3(reference)
  Demux2/1 -> PI-DT-Estimated d/2(reference)
  iIdq*/1 -> Demux2/1
  Demux3/1 -> PI-DT-Estimated d/3(initial)
  Demux3/2 -> PI-DT-Estimated q/2(initial)
  PI-DT-Estimated q/1(Out) -> sum_q/2
  vdq/1 -> Demux3/1
  PI-DT-Estimated d/1(Out) -> sum_d/1
  Mux/1 -> vidq*/1
  Demux1/2 -> wLq/1, PI-DT-Estimated q/1(actual)
  Demux1/1 -> PI-DT-Estimated d/4(actual), wLd/1
  iIdq/1 -> Demux1/1
  sum_q/1 -> Mux/2
  sum_d/1 -> Mux/1
  enable/1 -> Product/3, PI-DT-Estimated d/1(enable), Product1/3, PI-DT-Estimated q/4(enable)

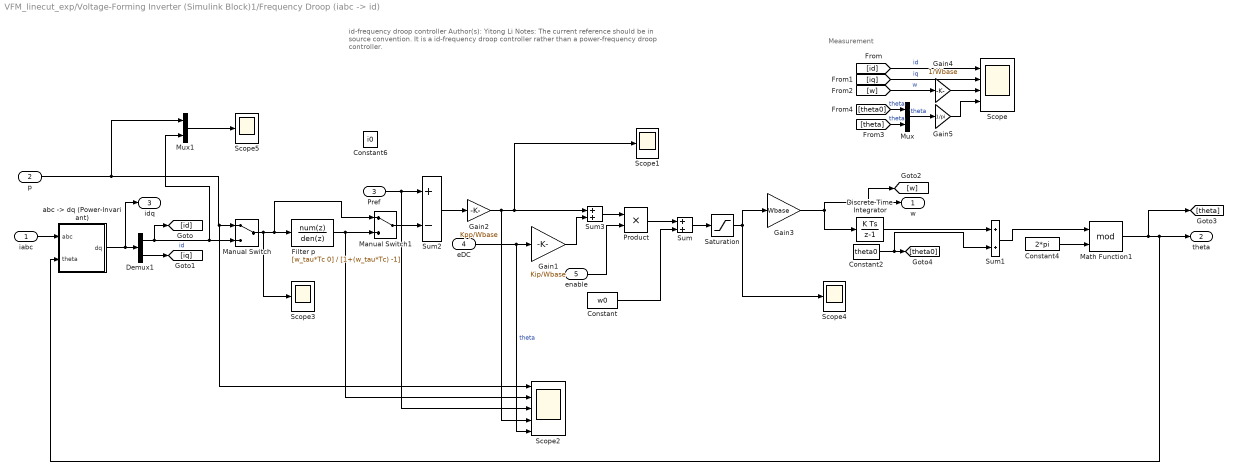
== system VFM_linecut_exp/Voltage-Forming Inverter (Simulink Block)1/Frequency Droop (iabc -> id) ==
  note: Measurement
  note: id-frequency droop controller
      |
      | Author(s): Yitong Li
      |
      | Notes:
      |
      | The current reference should be in source convention.
      |
      | It is a id-frequency droop controller rather than a power-frequency droop controller.
  iabc : Inport  SampleTime=Tc
  p : Inport  Port=2  SampleTime=Tc
  Pref : Inport  Port=3  SampleTime=Tc
  eDC : Inport  Port=4  SampleTime=Tc
  enable : Inport  Port=5  SampleTime=Tc
  Constant : Constant  Value=w0
  Constant2 : Constant  Value=theta0
  Constant4 : Constant  Value=2*pi
  Constant6 : Constant  Value=i0
  Demux1 : Demux  Outputs=2
  Discrete-Time Integrator : DiscreteIntegrator  SampleTime=Tc  ICPrevOutput=DiscIntNeverNeededParam  ICPrevScaledInput=DiscIntNeverNeededParam
  Filter p : DiscreteTransferFcn  LoadFcn=dspblkCoreblockFVToolHelper(gcbh,'load');  Numerator=[w_tau*Tc 0]  Denominator=[1+(w_tau*Tc) -1]  SampleTime=Tc
      settings: CopyFcn=dspblkCoreblockFVToolHelper(gcbh,'copy');  DeleteFcn=dspblkCoreblockFVToolHelper(gcbh,'close');  ModelCloseFcn=dspblkCoreblockFVToolHelper(gcbh,'close');  PreSaveFcn=dspblkCoreblockFVToolHelper(gcbh,'presave');  PostSaveFcn=dspblkCoreblockFVToolHelper(gcbh,'postsave');  CloseFcn=dspblkCoreblockFVToolHelper(gcbh,'close');
  Gain1 : Gain  Gain=Kip/Wbase
  Gain2 : Gain  Gain=Kpp/Wbase
  Gain3 : Gain  Gain=Wbase
  Gain4 : Gain  Gain=1/Wbase
  Gain5 : Gain  Gain=1/pi
  Manual Switch : ManualSwitch
  Manual Switch1 : ManualSwitch
  Math Function1 : Math  Operator=mod  SignedPower=on
  Mux : Mux  Inputs=2
  Mux1 : Mux  Inputs=2
  Product : Product
  Saturation : Saturate  UpperLimit=2  LowerLimit=-2
  Scope : Scope  NumInputPorts=4
      settings: ActiveDisplayYMinimum=-0.01955  ActiveDisplayYMaximum=0.17599
  Scope{1,3..5} (4 alike) : Scope
      Scope1 settings: ActiveDisplayYMinimum=-1.47341  ActiveDisplayYMaximum=1.22726  DataLoggingDecimation=10  DataLoggingVariableName=ScopeData2
      Scope3 settings: ActiveDisplayYMinimum=-4.53939  ActiveDisplayYMaximum=8.55763  DataLoggingDecimation=10  DataLoggingVariableName=ScopeData12
      Scope4 settings: ActiveDisplayYMinimum=-0.58842  ActiveDisplayYMaximum=2.08935  DataLoggingDecimation=10  DataLoggingVariableName=ScopeData13
      Scope5 settings: ActiveDisplayYMinimum=0.06721  ActiveDisplayYMaximum=3.86162  DataLoggingDecimation=10
  Scope2 : Scope  NumInputPorts=5
      settings: ActiveDisplayYMinimum=-0.96451219206720662  ActiveDisplayYMaximum=3.8373930452624223  DataLoggingVariableName=ScopeData2
  Sum : Sum
  Sum1 : Sum
  Sum2 : Sum  Inputs=+-
  Sum3 : Sum
  "abc -> dq (Power-Invariant)" : Subsystem  AncestorBlock=|
      | SimplusGT/abc -> dq
      | (Power-Invariant)
  w : Outport  SampleTime=Tc
  theta : Outport  Port=2  SampleTime=Tc
  idq : Outport  Port=3  SampleTime=Tc
  wires:
  Sum1/1 -> Math Function1/1
  Constant2/1 -> Sum1/2, [theta0]
  Discrete-Time Integrator/1 -> Sum1/1
  Constant/1 -> Sum/2
  "abc -> dq (Power-Invariant)"/1(dq) -> idq/1, Demux1/1
  Constant4/1 -> Math Function1/2
  iabc/1 -> "abc -> dq (Power-Invariant)"/1(abc)
  Sum2/1 -> Gain2/1
  Gain3/1 -> Discrete-Time Integrator/1, [w], w/1
  Demux1/1 -> Mux1/2, Manual Switch/2, [id]  "id"
  Gain5/1 -> Scope/4
  [iq] -> Scope/2  "iq"
  [theta0] -> Mux/1  "theta"
  [id] -> Scope/1  "id"
  Mux/1 -> Gain5/1  "theta"
  [theta] -> Mux/2  "theta"
  Demux1/2 -> [iq]
  [w] -> Gain4/1  "w"
  Gain4/1 -> Scope/3
  Sum/1 -> Saturation/1
  Saturation/1 -> Gain3/1, Scope4/1
  Manual Switch/1 -> Scope3/1, Filter p/1, Manual Switch1/1
  p/1 -> Mux1/1, Scope2/1, Manual Switch/1
  Filter p/1 -> Scope2/2, Manual Switch1/2
  Manual Switch1/1 -> Sum2/2
  Math Function1/1 -> "abc -> dq (Power-Invariant)"/2(theta), theta/1, [theta]
  Gain2/1 -> Sum3/1, Scope1/1, Scope2/4
  Mux1/1 -> Scope5/1
  Pref/1 -> Scope2/3, Sum2/1
  eDC/1 -> Scope2/5, Gain1/1  "theta"
  Gain1/1 -> Sum3/2
  Sum3/1 -> Product/1
  Product/1 -> Sum/1
  enable/1 -> Product/2
